simulink model "Pole_Placement_Jake"  (Simulink 8.9)
settings: Solver=VariableStepAuto  StartTime=0.0  StopTime=60  RelTol=1e-3
values from neighbouring files (symbols this model uses):
  K2 = 0.062    [Lab3_Pole_Placement_Integrator.m]
  K3 = 4.78    [Lab3_Pole_Placement_Integrator.m]
  T = 0.005    [Lab3_Pole_Placement_Integrator.m]
undefined symbols (not defined in the file or in its folder): Amplitude, C_den_inner, C_den_outer, C_num_inner, C_num_outer, Offset, P_inner
settings Model: Creator=joe  LastModifiedBy=jrampert
settings DataIOCC: LimitDataPoints=off  SaveFormat=Dataset  SignalLoggingSaveFormat=Dataset
settings DebuggingCC: UnderspecifiedInitializationDetection=Simplified  MergeDetectMultiDrivingBlocksExec=error  FcnCallInpInsideContextMsg=error  StateNameClashWarn=none  SFUnexpectedBacktrackingDiag=error  SFNoUnconditionalDefaultTransitionDiag=error
settings HardwareCC: ProdBitPerPointer=64  ProdBitPerSizeT=64  ProdBitPerPtrDiffT=64  ProdLargestAtomicFloat=Float  ProdIntDivRoundTo=Zero  ProdEndianess=LittleEndian  ProdWordSize=64  ProdHWDeviceType=Intel->x86-64 (Windows64)
settings ModelReferenceCC: PropagateSignalLabelsOutOfModel=on
settings GRTTargetCC: TargetLangStandard=C99 (ISO)  GeneratePreprocessorConditionals=Use local settings  CombineOutputUpdateFcns=on  GRTInterface=off
settings ConfigComp: CovMetricSettings=dwe  CovHtmlReporting=off  CovSaveCumulativeToWorkspaceVar=off  CovSaveSingleToWorkspaceVar=off  CovExternalEMLEnable=on

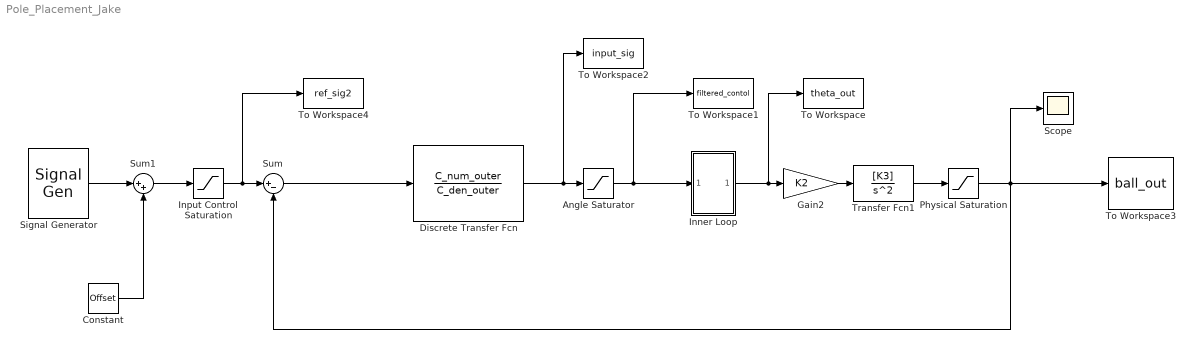
== system Pole_Placement_Jake ==
  Angle Saturator : Saturate  UpperLimit=0.785  LowerLimit=-0.785
  Constant : Constant  Value=Offset
  Discrete Transfer Fcn : DiscreteTransferFcn  Numerator=C_num_outer  Denominator=C_den_outer  SampleTime=T
  Gain2 : Gain  Gain=K2
  Inner Loop : Subsystem
  Input Control Saturation : Saturate  UpperLimit=0.417  LowerLimit=0
  Physical Saturation : Saturate  UpperLimit=0.417  LowerLimit=0
  Scope : Scope
  Signal Generator : SignalGenerator  WaveForm=square  Amplitude=Amplitude  Frequency=0.05
  Sum : Sum  Inputs=|+-
  Sum1 : Sum  Inputs=|++
  To Workspace : ToWorkspace  VariableName=theta_out  SaveFormat=Timeseries  SampleTime=-1
  To Workspace1 : ToWorkspace  VariableName=filtered_contol  SaveFormat=Timeseries  SampleTime=-1
  To Workspace2 : ToWorkspace  VariableName=input_sig  SaveFormat=Timeseries  SampleTime=-1
  To Workspace3 : ToWorkspace  VariableName=ball_out  SaveFormat=Timeseries  SampleTime=-1
  To Workspace4 : ToWorkspace  VariableName=ref_sig2  SaveFormat=Timeseries  SampleTime=-1
  Transfer Fcn1 : TransferFcn  Numerator=[K3]  Denominator=[1 0 0]
  wires:
  Discrete Transfer Fcn/1 -> To Workspace2/1, Angle Saturator/1
  Angle Saturator/1 -> To Workspace1/1, Inner Loop/1(In1)
  Sum/1 -> Discrete Transfer Fcn/1
  Input Control Saturation/1 -> To Workspace4/1, Sum/1
  Gain2/1 -> Transfer Fcn1/1
  Inner Loop/1(Out1) -> To Workspace/1, Gain2/1
  Transfer Fcn1/1 -> Physical Saturation/1
  Signal Generator/1 -> Sum1/1
  Sum1/1 -> Input Control Saturation/1
  Constant/1 -> Sum1/2
  Physical Saturation/1 -> Sum/2, To Workspace3/1, Scope/1

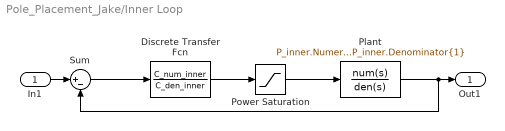
== system Pole_Placement_Jake/Inner Loop ==
  In1 : Inport
  Discrete Transfer Fcn : DiscreteTransferFcn  Numerator=C_num_inner  Denominator=C_den_inner
  Plant : TransferFcn  Numerator=P_inner.Numerator{1}  Denominator=P_inner.Denominator{1}
  Power Saturation : Saturate  UpperLimit=6  LowerLimit=-6
  Sum : Sum  Inputs=|+-
  Out1 : Outport
  wires:
  In1/1 -> Sum/1
  Plant/1 -> Sum/2, Out1/1
  Sum/1 -> Discrete Transfer Fcn/1
  Discrete Transfer Fcn/1 -> Power Saturation/1
  Power Saturation/1 -> Plant/1
